simulink model "Fliehkraft"  (R2022a)
settings: Solver=FixedStepAuto  StartTime=0.0  StopTime=10.0  FixedStep=0.001  RelTol=1e-3
values from neighbouring files (symbols this model uses):
  cr = 0.05    [Flieh.m]
  g = 9.81    [Flieh.m]
  l = 0.1    [Flieh.m]
  m = 0.5    [Flieh.m]
  rp = 0.01    [Flieh.m]
settings Model: Creator=JumpStart  LastModifiedBy=JumpStart

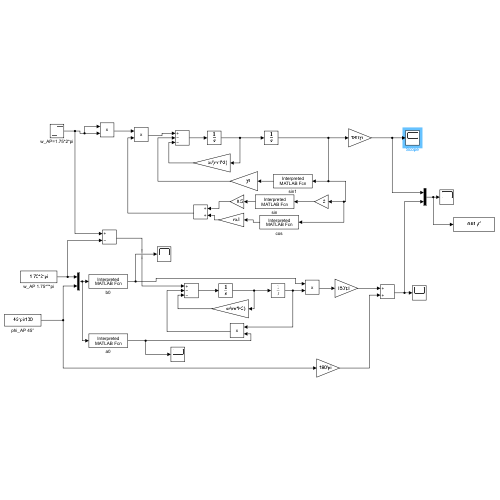
[thumbnail: Simulink's stored preview of the top-level diagram]
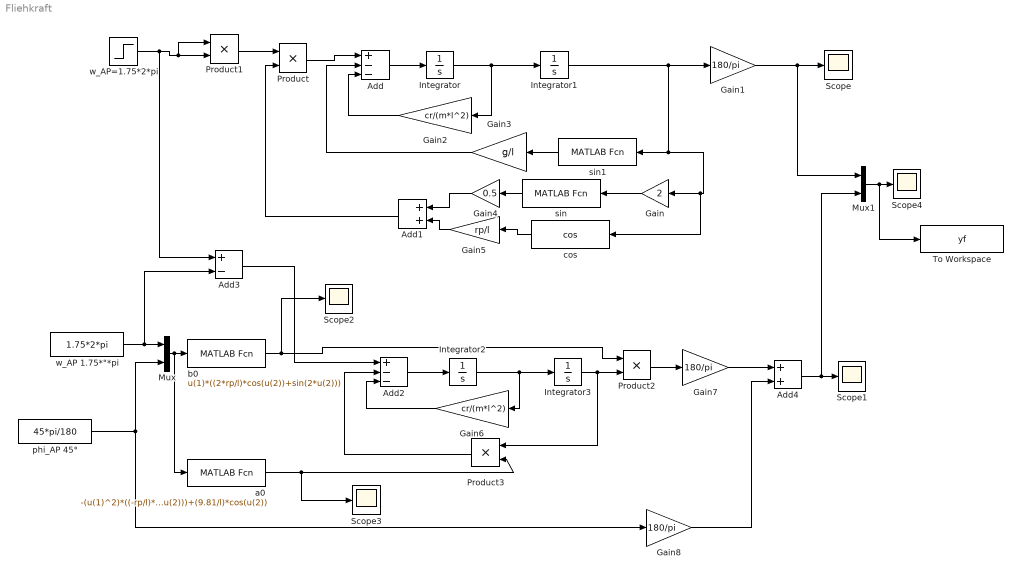
== system Fliehkraft ==
  Add : Sum  Inputs=+--
  Add1 : Sum
  Add2 : Sum  Inputs=+--
  Add3 : Sum  Inputs=+-
  Add4 : Sum
  Gain : Gain  Gain=2
  Gain1 : Gain  Gain=180/pi
  Gain2 : Gain  Gain=cr/(m*l^2)
  Gain3 : Gain  Gain=g/l
  Gain4 : Gain  Gain=0.5
  Gain5 : Gain  Gain=rp/l
  Gain6 : Gain  Gain=cr/(m*l^2)
  Gain7 : Gain  Gain=180/pi
  Gain8 : Gain  Gain=180/pi
  Integrator{,1..3} (4 alike) : Integrator
  Mux : Mux  Inputs=2
  Mux1 : Mux  Inputs=2
  Product{,1..3} (4 alike) : Product
  Scope{,1..4} (5 alike) : Scope
  To Workspace : ToWorkspace  VariableName=yf  SampleTime=-1
      settings: Save2DSignal=2-D array (concatenate along first dimension)
  a0 : MATLABFcn  MATLABFcn=-(u(1)^2)*((-rp/l)*sin(u(2))+cos(2*u(2)))+(9.81/l)*cos(u(2))
  b0 : MATLABFcn  MATLABFcn=u(1)*((2*rp/l)*cos(u(2))+sin(2*u(2)))
  cos : MATLABFcn  MATLABFcn=cos
  phi_AP 45° : Constant  Value=45*pi/180
  sin : MATLABFcn
  sin1 : MATLABFcn
  "w_AP 1.75*\"*pi" : Constant  Value=1.75*2*pi
  w_AP=1.75*2*pi : Step  Time=5  Before=1.75*2*pi  After=3*2*pi  SampleTime=0
  wires:
  Gain2/1 -> Add/3
  Gain3/1 -> Add/2
  sin1/1 -> Gain3/1
  Gain/1 -> sin/1
  sin/1 -> Gain4/1
  Gain4/1 -> Add1/1
  cos/1 -> Gain5/1
  Gain5/1 -> Add1/2
  Add1/1 -> Product/2
  Product/1 -> Add/1
  Product1/1 -> Product/1
  w_AP=1.75*2*pi/1 -> Add3/1, Product1/1, Product1/2
  Add/1 -> Integrator/1
  Integrator/1 -> Integrator1/1, Gain2/1
  Integrator1/1 -> Gain1/1, cos/1, Gain/1, sin1/1
  Gain1/1 -> Mux1/1, Scope/1
  "w_AP 1.75*\"*pi"/1 -> Add3/2, Mux/1
  phi_AP 45°/1 -> Gain8/1, Mux/2
  Mux/1 -> a0/1, b0/1
  b0/1 -> Scope2/1, Product2/1
  Integrator2/1 -> Gain6/1, Integrator3/1
  Add2/1 -> Integrator2/1
  Gain6/1 -> Add2/3
  Integrator3/1 -> Product3/1, Product2/2
  Product2/1 -> Gain7/1
  Product3/1 -> Add2/2
  a0/1 -> Scope3/1, Product3/2
  Add3/1 -> Add2/1
  Gain7/1 -> Add4/1
  Gain8/1 -> Add4/2
  Add4/1 -> Mux1/2, Scope1/1
  Mux1/1 -> To Workspace/1, Scope4/1
